simulink model "main_state_v3"  (R2021b)
settings: Solver=VariableStepAuto  StartTime=0.0  StopTime=inf  RelTol=1e-3
undefined symbols (not defined in the file): X, Y, Z
libraries: sm_lib x35, nesl_utility x19, simulink x11, fl_lib x6, ee_lib x3, slpidlib x1
(part 1 of 3)
settings Model: Creator=nose  LastModifiedBy=User

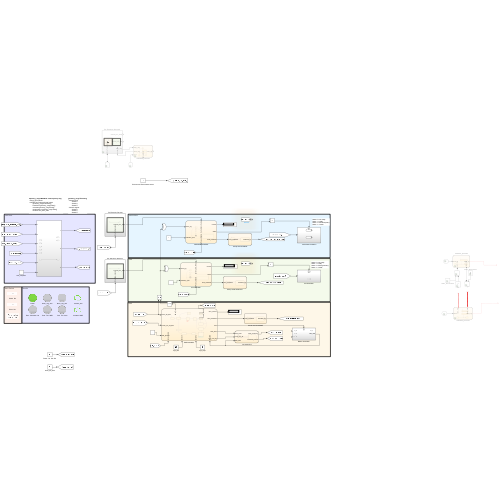
[thumbnail: Simulink's stored preview of the top-level diagram]
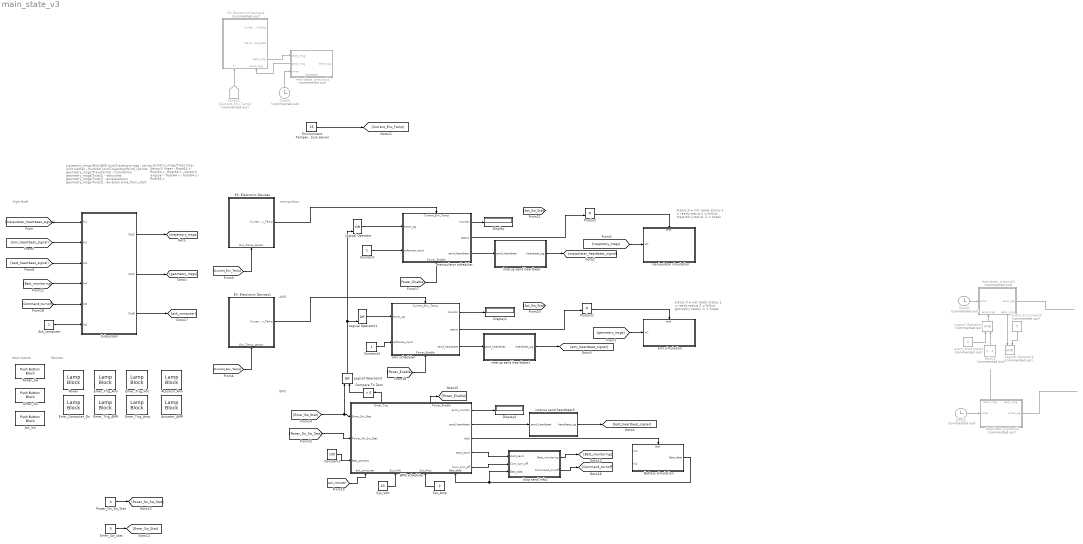
== system main_state_v3 ==
  note: geometry_msgs/Twist.msg
      | - Vector3 linear
      | - float64 x
      | - float64 y
      | - float64 z
      | - Vector3 angular
      | - float64 x
      | - float64 y
      | - float64 z
  note: trajectory_msgs/MultiDOF JointTrajectory.msg
      | - string [] joint names
      | - multidof jointTrajectoryPoint[] points
      | - geometry_msgs/Transform[]
      | - transforms geometry_msgs/Twist[]
      | - velocities geometry_msgs/Twist[]
      | - accelerations geometry_msgs/Twist[]
      | - duration time_from_start
  note: Monitor
  note: Main Switch
  note: status 0 = not ready
      | status 1 = ready
      | status 2 = follow trajectory
      | status -1 = break
  note: BMS
  note: high-level
  note: AMR
  note: manipulator
  note: status 0 = not ready
      | status 1 = ready
      | status 2 = follow geometry
      | status -1 = break
  Ack_computer : Constant
  Act_Sw : PushButtonBlock  ButtonType=Latch  OffValue=0.000000
  Actuator_AMR : LampBlock  LabelPosition=Hide  Icon=Engine
  Actuator_Arm : LampBlock  LabelPosition=Hide  Icon=Engine
  BMS scheduler : Stateflow chart  TreatAsAtomicUnit=on
      settings: PortSchema="{\"entries\":[{\"content\":{\"sides\":[{\"content\":{\"connectorIds\":[\"In3\",\"In2\",\"In4\"]},\"type\":\"ConnectorPlacement.EquallySpacedRectSide\",\"uuid\":\"e14584fa-6c70-433d-b2da-38d1197773c6\"},{\"content\":{\"connectorIds\":[\"Out4\",\"Out7\",\"Out2\",\"Out1\",\"Out5\"],\"side\":\"RIGHT\"},\"type\":\"ConnectorPlacement.EquallySpacedRectSide\",\"uuid\":\"c0129660-3601-4a2d-a8be-6a057e5db4e4\"},{\"content\":{\"connectorIds\":[\"Out6\",\"Out3\"],\"side\":\"TOP\"},\"type\":\"ConnectorPlacement.EquallySpacedRectSide\",\"uuid\":\"ad450ee9-aa73-4b1e-81ef-c89dc6269e7d\"},{\"content\":{\"connectorIds\":[\"In1\",\"In6\",\"In7\",\"In5\"],\"side\":\"BOTTOM\"},\"type\":\"ConnectorPlacement.EquallySpacedRectSide\",\"uuid\":\"07d48c63-9776-4fdb-82a7-d3bb7c8bd27e\"}]},\"type\":\"ConnectorPlacement.EquallySpacedConnector\",\"uuid\":\"cc336b9e-cb49-4b3a-8aca-cb2cce9a2aaf\"}],\"packageUris\":[\"http://schema.mathworks.com/mf0/Connector/R2020b\"],\"version\":\"1.0\"}"
  Battery simulation : Subsystem
      settings: PortSchema="{\"entries\":[{\"content\":{\"sides\":[{\"content\":{\"connectorIds\":[\"In1\",\"In2\"]},\"type\":\"ConnectorPlacement.EquallySpacedRectSide\",\"uuid\":\"e14584fa-6c70-433d-b2da-38d1197773c6\"},{\"content\":{\"connectorIds\":[\"Out1\"],\"side\":\"RIGHT\"},\"type\":\"ConnectorPlacement.EquallySpacedRectSide\",\"uuid\":\"c0129660-3601-4a2d-a8be-6a057e5db4e4\"},{\"content\":{\"connectorIds\":[\"In3\"],\"side\":\"TOP\"},\"type\":\"ConnectorPlacement.EquallySpacedRectSide\",\"uuid\":\"ad450ee9-aa73-4b1e-81ef-c89dc6269e7d\"}]},\"type\":\"ConnectorPlacement.EquallySpacedConnector\",\"uuid\":\"cc336b9e-cb49-4b3a-8aca-cb2cce9a2aaf\"}],\"packageUris\":[\"http://schema.mathworks.com/mf0/Connector/R2020b\"],\"version\":\"1.0\"}"
  Clock2 : Clock  Commented=on
  Clock3 : Clock  Commented=on
  Clock5 : Clock  Commented=on
  Compare To Zero : simulink/Logic and Bit Operations/Compare To Zero  relop=>  OutDataTypeStr=boolean
  Constant : Constant
  Constant2 : Constant
  Constant3 : Constant  Value=100
  Delay1 : Delay  Commented=on  DelayLength=1
  Display : Display
  Display1 : Display
  Display2 : Display
  EX. Electronic Devices : Subsystem
      settings: PortSchema="{\"entries\":[{\"content\":{\"sides\":[{\"content\":{\"connectorIds\":[]},\"type\":\"ConnectorPlacement.EquallySpacedRectSide\",\"uuid\":\"2093f37f-91bf-4439-a287-00f2f1b8dec3\"},{\"content\":{\"connectorIds\":[\"Out1\"],\"side\":\"RIGHT\"},\"type\":\"ConnectorPlacement.EquallySpacedRectSide\",\"uuid\":\"bc710c56-ac77-428e-a7cb-e88f032cce03\"},{\"content\":{\"connectorIds\":[],\"side\":\"TOP\"},\"type\":\"ConnectorPlacement.EquallySpacedRectSide\",\"uuid\":\"1d82479b-6b77-4f2a-b8f4-b2e895a94223\"},{\"content\":{\"connectorIds\":[\"In1\"],\"side\":\"BOTTOM\"},\"type\":\"ConnectorPlacement.EquallySpacedRectSide\",\"uuid\":\"16a89f62-a8a8-40ba-a530-69de77f13aa0\"}]},\"type\":\"ConnectorPlacement.EquallySpacedConnector\",\"uuid\":\"46f96c33-35b8-4147-a04e-6429fc761b64\"}],\"packageUris\":[\"http://schema.mathworks.com/mf0/Connector/R2020b\"],\"version\":\"1.0\"}"
  EX. Electronic Devices1 : Subsystem
      settings: PortSchema="{\"entries\":[{\"content\":{\"sides\":[{\"content\":{\"connectorIds\":[]},\"type\":\"ConnectorPlacement.EquallySpacedRectSide\",\"uuid\":\"2093f37f-91bf-4439-a287-00f2f1b8dec3\"},{\"content\":{\"connectorIds\":[\"Out1\"],\"side\":\"RIGHT\"},\"type\":\"ConnectorPlacement.EquallySpacedRectSide\",\"uuid\":\"bc710c56-ac77-428e-a7cb-e88f032cce03\"},{\"content\":{\"connectorIds\":[],\"side\":\"TOP\"},\"type\":\"ConnectorPlacement.EquallySpacedRectSide\",\"uuid\":\"1d82479b-6b77-4f2a-b8f4-b2e895a94223\"},{\"content\":{\"connectorIds\":[\"In1\"],\"side\":\"BOTTOM\"},\"type\":\"ConnectorPlacement.EquallySpacedRectSide\",\"uuid\":\"16a89f62-a8a8-40ba-a530-69de77f13aa0\"}]},\"type\":\"ConnectorPlacement.EquallySpacedConnector\",\"uuid\":\"46f96c33-35b8-4147-a04e-6429fc761b64\"}],\"packageUris\":[\"http://schema.mathworks.com/mf0/Connector/R2020b\"],\"version\":\"1.0\"}"
  EX. Electronic Devices2 : Subsystem  Commented=on
      settings: PortSchema="{\"entries\":[{\"content\":{\"sides\":[{\"content\":{\"connectorIds\":[]},\"type\":\"ConnectorPlacement.EquallySpacedRectSide\",\"uuid\":\"2093f37f-91bf-4439-a287-00f2f1b8dec3\"},{\"content\":{\"connectorIds\":[\"Out1\",\"Out2\",\"Out3\"],\"side\":\"RIGHT\"},\"type\":\"ConnectorPlacement.EquallySpacedRectSide\",\"uuid\":\"bc710c56-ac77-428e-a7cb-e88f032cce03\"},{\"content\":{\"connectorIds\":[],\"side\":\"TOP\"},\"type\":\"ConnectorPlacement.EquallySpacedRectSide\",\"uuid\":\"1d82479b-6b77-4f2a-b8f4-b2e895a94223\"},{\"content\":{\"connectorIds\":[\"In1\",\"In2\"],\"side\":\"BOTTOM\"},\"type\":\"ConnectorPlacement.EquallySpacedRectSide\",\"uuid\":\"16a89f62-a8a8-40ba-a530-69de77f13aa0\"}]},\"type\":\"ConnectorPlacement.EquallySpacedConnector\",\"uuid\":\"46f96c33-35b8-4147-a04e-6429fc761b64\"}],\"packageUris\":[\"http://schema.mathworks.com/mf0/Connector/R2020b\"],\"version\":\"1.0\"}"
  Emer_Sw : PushButtonBlock  ButtonType=Latch  OffValue=0.000000
  Emer_Sw_Stat : Constant  Value=0
  Emer_Trig_AMR : LampBlock  LabelPosition=Hide
  Emer_Trig_Amp : LampBlock  LabelPosition=Hide
  Emer_Trig_Arm : LampBlock  LabelPosition=Hide
  Emer_Trig_Volt : LampBlock  LabelPosition=Hide
  Environment Temperature sensor : Constant  Value=25
  Error_Computer_On : LampBlock  LabelPosition=Hide
  From22 : From  Commented=on  GotoTag=Current_Env_Temp
  Heartbeat_protocol2 : Stateflow chart  Commented=on  TreatAsAtomicUnit=on
      settings: PortSchema="{\"entries\":[{\"content\":{\"sides\":[{\"content\":{\"connectorIds\":[\"In1\"]},\"type\":\"ConnectorPlacement.EquallySpacedRectSide\",\"uuid\":\"669ad136-449b-4cce-8c88-f277646368db\"},{\"content\":{\"connectorIds\":[\"Out2\"],\"side\":\"RIGHT\"},\"type\":\"ConnectorPlacement.EquallySpacedRectSide\",\"uuid\":\"85d872e5-bd76-461e-b542-94d453191651\"},{\"content\":{\"connectorIds\":[],\"side\":\"TOP\"},\"type\":\"ConnectorPlacement.EquallySpacedRectSide\",\"uuid\":\"fd46d66d-a650-417c-aa37-2d0cce1d3427\"},{\"content\":{\"connectorIds\":[\"In2\",\"Out1\"],\"side\":\"BOTTOM\"},\"type\":\"ConnectorPlacement.EquallySpacedRectSide\",\"uuid\":\"b50bf124-1357-4fec-a689-784ede394cd4\"}]},\"type\":\"ConnectorPlacement.EquallySpacedConnector\",\"uuid\":\"8f3d29fd-8071-4b41-baf0-05db73c814ac\"}],\"packageUris\":[\"http://schema.mathworks.com/mf0/Connector/R2020b\"],\"version\":\"1.0\"}"
  Heartbeat_protocol3 : Stateflow chart  Commented=on  TreatAsAtomicUnit=on
      settings: PortSchema="{\"entries\":[{\"content\":{\"sides\":[{\"content\":{\"connectorIds\":[\"In1\"]},\"type\":\"ConnectorPlacement.EquallySpacedRectSide\",\"uuid\":\"55ab65ce-874e-4ed3-8904-faffec9acc87\"},{\"content\":{\"connectorIds\":[\"Out2\"],\"side\":\"RIGHT\"},\"type\":\"ConnectorPlacement.EquallySpacedRectSide\",\"uuid\":\"0d2cd230-18ea-4b79-8380-304b366a5a71\"},{\"content\":{\"connectorIds\":[\"Out1\",\"In2\"],\"side\":\"TOP\"},\"type\":\"ConnectorPlacement.EquallySpacedRectSide\",\"uuid\":\"c9fbaa84-af0b-41d8-82b6-91783628c705\"}]},\"type\":\"ConnectorPlacement.EquallySpacedConnector\",\"uuid\":\"c6b505fd-b4aa-4ed2-9cf9-f91253423c66\"}],\"packageUris\":[\"http://schema.mathworks.com/mf0/Connector/R2020b\"],\"version\":\"1.0\"}"
  Heartbeat_protocol4 : Stateflow chart  Commented=on  TreatAsAtomicUnit=on
      settings: PortSchema="{\"entries\":[{\"content\":{\"sides\":[{\"content\":{\"connectorIds\":[\"In3\",\"Out1\",\"In2\"]},\"type\":\"ConnectorPlacement.EquallySpacedRectSide\",\"uuid\":\"55ab65ce-874e-4ed3-8904-faffec9acc87\"},{\"content\":{\"connectorIds\":[\"Out2\"],\"side\":\"RIGHT\"},\"type\":\"ConnectorPlacement.EquallySpacedRectSide\",\"uuid\":\"0d2cd230-18ea-4b79-8380-304b366a5a71\"},{\"content\":{\"connectorIds\":[],\"side\":\"TOP\"},\"type\":\"ConnectorPlacement.EquallySpacedRectSide\",\"uuid\":\"c9fbaa84-af0b-41d8-82b6-91783628c705\"},{\"content\":{\"connectorIds\":[\"In1\"],\"side\":\"BOTTOM\"},\"type\":\"ConnectorPlacement.EquallySpacedRectSide\",\"uuid\":\"5c6b53c8-9610-4554-8826-ed179a52c636\"}]},\"type\":\"ConnectorPlacement.EquallySpacedConnector\",\"uuid\":\"c6b505fd-b4aa-4ed2-9cf9-f91253423c66\"}],\"packageUris\":[\"http://schema.mathworks.com/mf0/Connector/R2020b\"],\"version\":\"1.0\"}"
  Logical Operator : Logic  Operator=OR  Inputs=3  IconShape=distinctive  AllPortsSameDT=off  OutDataTypeStr=boolean
  Logical Operator1 : Logic  Operator=OR  Inputs=3  IconShape=distinctive  AllPortsSameDT=off  OutDataTypeStr=boolean
  Logical Operator2 : Logic  Operator=OR  AllPortsSameDT=off  OutDataTypeStr=boolean
  Logical Operator3 : Logic  Commented=on  AllPortsSameDT=off  OutDataTypeStr=boolean
  Logical Operator4 : Logic  Commented=on  AllPortsSameDT=off  OutDataTypeStr=boolean
  Power : LampBlock  LabelPosition=Hide
  Power_On_Sw_Stat : Constant  Value=0
  Power_Sw : PushButtonBlock  OffValue=0.000000
  Product : Product
  Product1 : Product
  Subsystem : Subsystem
  Sys_Amp : Constant  Value=2
  Sys_Volt : Constant  Value=20
  amr scheduler : Stateflow chart  TreatAsAtomicUnit=on
      settings: PortSchema="{\"entries\":[{\"content\":{\"sides\":[{\"content\":{\"connectorIds\":[\"In3\",\"In4\"]},\"type\":\"ConnectorPlacement.EquallySpacedRectSide\",\"uuid\":\"e14584fa-6c70-433d-b2da-38d1197773c6\"},{\"content\":{\"connectorIds\":[\"Out1\",\"Out2\",\"Out3\"],\"side\":\"RIGHT\"},\"type\":\"ConnectorPlacement.EquallySpacedRectSide\",\"uuid\":\"c0129660-3601-4a2d-a8be-6a057e5db4e4\"},{\"content\":{\"connectorIds\":[\"In2\"],\"side\":\"TOP\"},\"type\":\"ConnectorPlacement.EquallySpacedRectSide\",\"uuid\":\"ad450ee9-aa73-4b1e-81ef-c89dc6269e7d\"},{\"content\":{\"connectorIds\":[\"In1\"],\"side\":\"BOTTOM\"},\"type\":\"ConnectorPlacement.EquallySpacedRectSide\",\"uuid\":\"ee7aab22-cd29-46c3-88a9-d3e335dac3e8\"}]},\"type\":\"ConnectorPlacement.EquallySpacedConnector\",\"uuid\":\"cc336b9e-cb49-4b3a-8aca-cb2cce9a2aaf\"}],\"packageUris\":[\"http://schema.mathworks.com/mf0/Connector/R2020b\"],\"version\":\"1.0\"}"
  amr simulation : Subsystem
      settings: PortSchema="{\"entries\":[{\"content\":{\"sides\":[{\"content\":{\"connectorIds\":[\"In1\"]},\"type\":\"ConnectorPlacement.EquallySpacedRectSide\",\"uuid\":\"e14584fa-6c70-433d-b2da-38d1197773c6\"},{\"content\":{\"connectorIds\":[],\"side\":\"RIGHT\"},\"type\":\"ConnectorPlacement.EquallySpacedRectSide\",\"uuid\":\"c0129660-3601-4a2d-a8be-6a057e5db4e4\"},{\"content\":{\"connectorIds\":[\"In2\"],\"side\":\"TOP\"},\"type\":\"ConnectorPlacement.EquallySpacedRectSide\",\"uuid\":\"ad450ee9-aa73-4b1e-81ef-c89dc6269e7d\"}]},\"type\":\"ConnectorPlacement.EquallySpacedConnector\",\"uuid\":\"cc336b9e-cb49-4b3a-8aca-cb2cce9a2aaf\"}],\"packageUris\":[\"http://schema.mathworks.com/mf0/Connector/R2020b\"],\"version\":\"1.0\"}"
  exam_disconnect2 : Constant  Commented=on  Value=0
  exam_disconnect3 : Constant  Commented=on  Value=0
  interup send heartbeat : Stateflow chart  TreatAsAtomicUnit=on
  interup send heartbeat1 : Stateflow chart  TreatAsAtomicUnit=on
  interup send heartbeat3 : Stateflow chart  TreatAsAtomicUnit=on
  loop send info2 : Stateflow chart  TreatAsAtomicUnit=on
  manipulator scheduler : Stateflow chart  TreatAsAtomicUnit=on
      settings: PortSchema="{\"entries\":[{\"content\":{\"sides\":[{\"content\":{\"connectorIds\":[\"In3\",\"In4\"]},\"type\":\"ConnectorPlacement.EquallySpacedRectSide\",\"uuid\":\"e14584fa-6c70-433d-b2da-38d1197773c6\"},{\"content\":{\"connectorIds\":[\"Out2\",\"Out1\",\"Out3\"],\"side\":\"RIGHT\"},\"type\":\"ConnectorPlacement.EquallySpacedRectSide\",\"uuid\":\"c0129660-3601-4a2d-a8be-6a057e5db4e4\"},{\"content\":{\"connectorIds\":[\"In2\"],\"side\":\"TOP\"},\"type\":\"ConnectorPlacement.EquallySpacedRectSide\",\"uuid\":\"ad450ee9-aa73-4b1e-81ef-c89dc6269e7d\"},{\"content\":{\"connectorIds\":[\"In1\"],\"side\":\"BOTTOM\"},\"type\":\"ConnectorPlacement.EquallySpacedRectSide\",\"uuid\":\"918673b1-c838-461d-b96b-adbd07e06c61\"}]},\"type\":\"ConnectorPlacement.EquallySpacedConnector\",\"uuid\":\"cc336b9e-cb49-4b3a-8aca-cb2cce9a2aaf\"}],\"packageUris\":[\"http://schema.mathworks.com/mf0/Connector/R2020b\"],\"version\":\"1.0\"}"
  manipulator simulation : Subsystem
      settings: PortSchema="{\"entries\":[{\"content\":{\"sides\":[{\"content\":{\"connectorIds\":[\"In1\"]},\"type\":\"ConnectorPlacement.EquallySpacedRectSide\",\"uuid\":\"80f1c3ab-f726-46f3-9980-68f35c05e058\"},{\"content\":{\"connectorIds\":[],\"side\":\"RIGHT\"},\"type\":\"ConnectorPlacement.EquallySpacedRectSide\",\"uuid\":\"8613bb6a-65ca-45e7-9d44-92dca48eb7bb\"},{\"content\":{\"connectorIds\":[\"In2\"],\"side\":\"TOP\"},\"type\":\"ConnectorPlacement.EquallySpacedRectSide\",\"uuid\":\"e26f3b3a-06b4-4643-8203-7aff778e7067\"}]},\"type\":\"ConnectorPlacement.EquallySpacedConnector\",\"uuid\":\"cedcd8d2-6fb7-4e87-9ef3-c550760e1c47\"}],\"packageUris\":[\"http://schema.mathworks.com/mf0/Connector/R2020b\"],\"version\":\"1.0\"}"
  wires:
  Constant/1 -> manipulator scheduler/4(software_input)
  amr scheduler/3(send_heartbeat) -> interup send heartbeat1/1(send_heartbeat)
  Subsystem/1(Out2) -> [trajectory_msgs]
  Subsystem/2(Out1) -> [geometry_msgs]
  [maipulater_heartbeat_signal] -> Subsystem/1(In1)
  loop send info2/1(Batt_monitoring) -> [Batt_monitoring]
  [Batt_monitoring] -> Subsystem/4(In4)
  BMS scheduler/2(task) -> Battery simulation/3(task)
  Battery simulation/1(Batt_data) -> loop send info2/3(Batt_data), BMS scheduler/5(Batt_data)
  BMS scheduler/1(start_send) -> loop send info2/1(start_send)
  Constant3/1 -> BMS scheduler/4(Batt_percent)
  Heartbeat_protocol2/2(emer_sig) -> ?
  Delay1/1 -> Logical Operator3/2
  exam_disconnect3/1 -> Logical Operator4/2
  Logical Operator3/1 -> Heartbeat_protocol2/2(send_msg)
  exam_disconnect2/1 -> Logical Operator3/1
  Clock2/1 -> Heartbeat_protocol2/1(timer)
  Heartbeat_protocol2/1(reply_msg) -> Logical Operator4/1
  ? -> Heartbeat_protocol3/2(reply_msg)
  Heartbeat_protocol3/2(emer_sig) -> ?
  Clock3/1 -> Heartbeat_protocol3/1(timer)
  Heartbeat_protocol3/1(send_msg) -> ?
  Logical Operator/1 -> manipulator scheduler/3(emer_sig)
  Logical Operator1/1 -> amr scheduler/3(emer_sig)
  Environment Temperature sensor/1 -> [Current_Env_Temp]
  EX. Electronic Devices/1(Current_Env_Temp) -> manipulator scheduler/2(Current_Env_Temp)
  Emer_Sw_Stat/1 -> [Emer_Sw_Stat]
  [Emer_Sw_Stat] -> Logical Operator2/1, BMS scheduler/3(Emer_Sw_Stat)
  [Power_On_Sw_Stat] -> BMS scheduler/2(Power_On_Sw_Stat)
  BMS scheduler/3(Power_Enable) -> [Power_Enable]
  [Power_Enable] -> amr scheduler/1(Power_Enable)
  [Power_Enable] -> manipulator scheduler/1(Power_Enable)
  manipulator scheduler/2(monitor) -> Display/1
  amr scheduler/1(monitor) -> Display1/1
  [ack_computer] -> BMS scheduler/1(ack_computer)
  Power_On_Sw_Stat/1 -> [Power_On_Sw_Stat]
  BMS scheduler/5(Com_turn_off) -> loop send info2/2(Com_turn_off)
  loop send info2/2(Command_turnoff) -> [Command_turnoff]
  [Command_turnoff] -> Subsystem/5(In5)
  BMS scheduler/4(error_monitor) -> Display2/1
  Ack_computer/1 -> Subsystem/6(In6)
  Subsystem/3(Out8) -> [ack_computer]
  Sys_Volt/1 -> BMS scheduler/6(Sys_Volt)
  Sys_Amp/1 -> BMS scheduler/7(Sys_Amp)
  BMS scheduler/6(Emer_Trig) -> Compare To Zero/1
  Compare To Zero/1 -> Logical Operator2/2
  Logical Operator2/1 -> Logical Operator/3, Logical Operator1/3
  Product/1 -> manipulator simulation/2(task)
  manipulator scheduler/1(status) -> Product/2
  amr scheduler/2(status) -> Product1/2
  Product1/1 -> amr simulation/2(task)
  Clock5/1 -> Heartbeat_protocol4/2(timer)
  From22/1 -> EX. Electronic Devices2/1(Env_Temp_sensor)
  Heartbeat_protocol4/1(send_msg) -> EX. Electronic Devices2/2(send_msg)
  EX. Electronic Devices2/3(reply_msg) -> Heartbeat_protocol4/3(reply_msg)
  manipulator scheduler/3(send_heartbeat) -> interup send heartbeat/1(send_heartbeat)
  interup send heartbeat/1(heartbeat_sig) -> [maipulater_heartbeat_signal]
  EX. Electronic Devices1/1(Current_Env_Temp) -> amr scheduler/2(Current_Env_Temp)
  [Current_Env_Temp] -> EX. Electronic Devices/1(Env_Temp_sensor)
  [Current_Env_Temp] -> EX. Electronic Devices1/1(Env_Temp_sensor)
  interup send heartbeat1/1(heartbeat_sig) -> [amr_heartbeat_signal]
  Constant2/1 -> amr scheduler/4(software_input)
  [geometry_msgs] -> amr simulation/1(In1)
  [trajectory_msgs] -> manipulator simulation/1(In1)
  [amr_heartbeat_signal] -> Subsystem/2(In2)
  BMS scheduler/7(send_heartbeat) -> interup send heartbeat3/1(send_heartbeat)
  [batt_heartbeat_signal] -> Subsystem/3(In3)
  interup send heartbeat3/1(heartbeat_sig) -> [batt_heartbeat_signal]

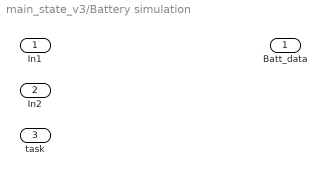
== system main_state_v3/Battery simulation ==
  In1 : Inport
  In2 : Inport  Port=2
  task : Inport  Port=3
  Batt_data : Outport

== system main_state_v3/EX. Electronic Devices ==
  note: Environment Temperature Warning (both over and under)
  Env_Temp_sensor : Inport
  Current_Env_Temp : Outport
  wires:
  Env_Temp_sensor/1 -> Current_Env_Temp/1

== system main_state_v3/EX. Electronic Devices1 ==
  note: Environment Temperature Warning (both over and under)
  Env_Temp_sensor : Inport
  Current_Env_Temp : Outport
  wires:
  Env_Temp_sensor/1 -> Current_Env_Temp/1

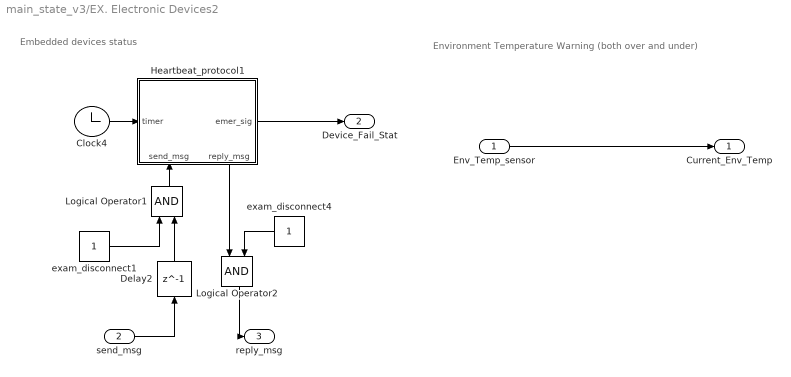
== system main_state_v3/EX. Electronic Devices2 ==
  note: Embedded devices status
  note: Environment Temperature Warning (both over and under)
  Env_Temp_sensor : Inport
  send_msg : Inport  Port=2
  Clock4 : Clock
  Delay2 : Delay  DelayLength=1
  Heartbeat_protocol1 : Stateflow chart  TreatAsAtomicUnit=on
      settings: PortSchema="{\"entries\":[{\"content\":{\"sides\":[{\"content\":{\"connectorIds\":[\"In1\"]},\"type\":\"ConnectorPlacement.EquallySpacedRectSide\",\"uuid\":\"669ad136-449b-4cce-8c88-f277646368db\"},{\"content\":{\"connectorIds\":[\"Out2\"],\"side\":\"RIGHT\"},\"type\":\"ConnectorPlacement.EquallySpacedRectSide\",\"uuid\":\"85d872e5-bd76-461e-b542-94d453191651\"},{\"content\":{\"connectorIds\":[],\"side\":\"TOP\"},\"type\":\"ConnectorPlacement.EquallySpacedRectSide\",\"uuid\":\"fd46d66d-a650-417c-aa37-2d0cce1d3427\"},{\"content\":{\"connectorIds\":[\"In2\",\"Out1\"],\"side\":\"BOTTOM\"},\"type\":\"ConnectorPlacement.EquallySpacedRectSide\",\"uuid\":\"b50bf124-1357-4fec-a689-784ede394cd4\"}]},\"type\":\"ConnectorPlacement.EquallySpacedConnector\",\"uuid\":\"8f3d29fd-8071-4b41-baf0-05db73c814ac\"}],\"packageUris\":[\"http://schema.mathworks.com/mf0/Connector/R2020b\"],\"version\":\"1.0\"}"
  Logical Operator1 : Logic  AllPortsSameDT=off  OutDataTypeStr=boolean
  Logical Operator2 : Logic  AllPortsSameDT=off  OutDataTypeStr=boolean
  exam_disconnect1 : Constant
  exam_disconnect4 : Constant
  Current_Env_Temp : Outport
  Device_Fail_Stat : Outport  Port=2
  reply_msg : Outport  Port=3
  wires:
  Env_Temp_sensor/1 -> Current_Env_Temp/1
  Logical Operator2/1 -> reply_msg/1
  Delay2/1 -> Logical Operator1/2
  exam_disconnect4/1 -> Logical Operator2/2
  Logical Operator1/1 -> Heartbeat_protocol1/2(send_msg)
  send_msg/1 -> Delay2/1
  Heartbeat_protocol1/2(emer_sig) -> Device_Fail_Stat/1
  Clock4/1 -> Heartbeat_protocol1/1(timer)
  Heartbeat_protocol1/1(reply_msg) -> Logical Operator2/1
  exam_disconnect1/1 -> Logical Operator1/1

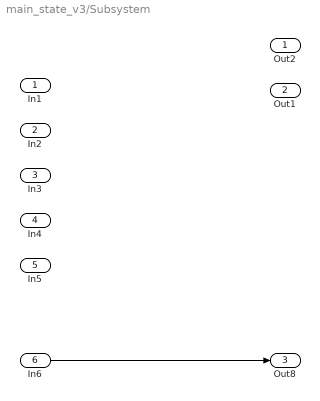
== system main_state_v3/Subsystem ==
  In1 : Inport
  In2 : Inport  Port=2
  In3 : Inport  Port=3
  In4 : Inport  Port=4
  In5 : Inport  Port=5
  In6 : Inport  Port=6
  Out2 : Outport
  Out1 : Outport  Port=2
  Out8 : Outport  Port=3
  wires:
  In6/1 -> Out8/1

== system main_state_v3/amr simulation ==
  In1 : Inport
  task : Inport  Port=2
